simulink model "Sis_Mecanico"  (R2025b)
settings: Solver=VariableStepAuto  StartTime=0.0  StopTime=2  RelTol=1e-3
libraries: fl_lib x7, nesl_utility x3
settings Model: Creator=Brayan Barragan  LastModifiedBy=Brayan Barragan

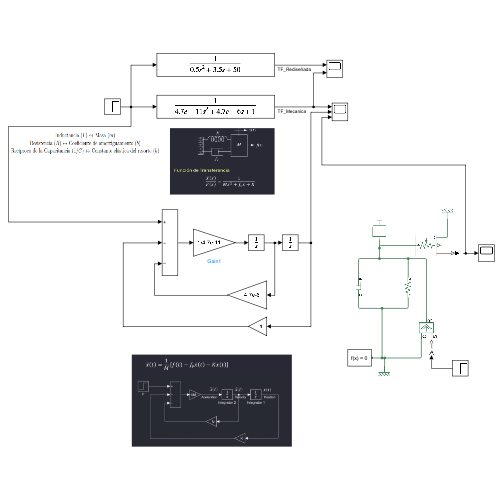
[thumbnail: Simulink's stored preview of the top-level diagram]
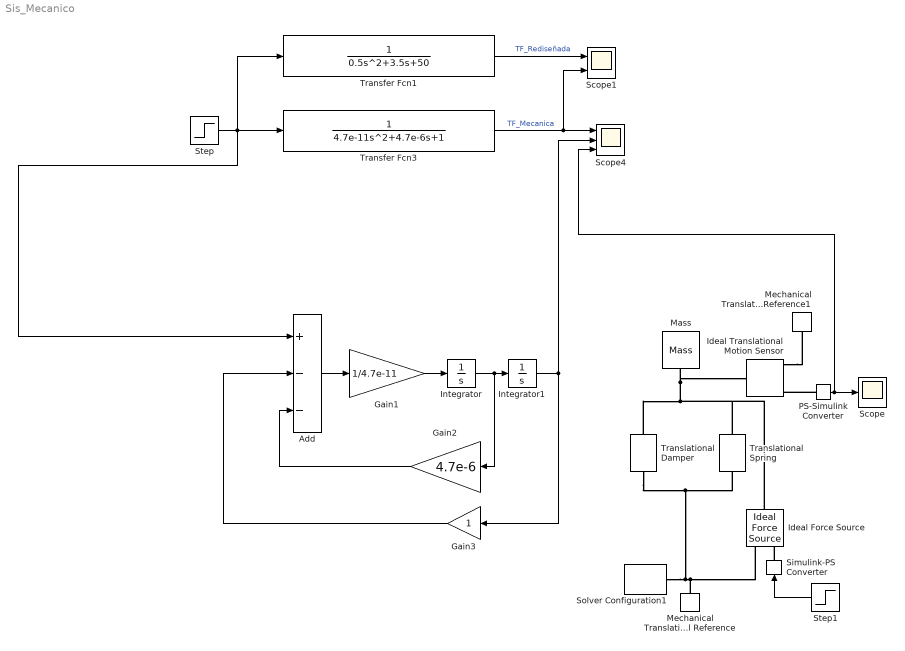
== system Sis_Mecanico ==
  Add : Sum  Inputs=+--
  Gain1 : Gain  Gain=1/4.7e-11
  Gain2 : Gain  Gain=4.7e-6
  Gain3 : Gain
  Ideal Force Source : fl_lib/Mechanical/Mechanical Sources/Ideal Force Source
  Ideal Translational Motion Sensor : fl_lib/Mechanical/Mechanical Sensors/Ideal Translational Motion Sensor  reference=foundation.enum.MeasurementReference.difference  acceleration_port=false  velocity_port=true  position_port=true  offset=0 m
  Integrator : Integrator
  Integrator1 : Integrator
  Mass : fl_lib/Mechanical/Translational Elements/Mass  mass=4.7e-11 kg  num_ports=foundation.enum.numPorts2.one  v_specify=off  v_priority=High  v=0 m/s  v_nominal_specify=off  v_nominal_value=1  v_nominal_unit=m/s  f_specify=off  f_priority=None  f=0 N  f_nominal_specify=off  f_nominal_value=1  f_nominal_unit=N
  Mechanical Translational Reference : fl_lib/Mechanical/Translational Elements/Mechanical Translational Reference
  Mechanical Translational Reference1 : fl_lib/Mechanical/Translational Elements/Mechanical Translational Reference
  PS-Simulink Converter : nesl_utility/PS-Simulink Converter  PhysicalDomain=network_engine_domain  SubClassName=ps_output  LeftPortType=input  RightPortType=output  PseudoPeriodic=off  Frequencies=[]  VectorFormat=inherit  Unit=inherit  AffineConversion=off
  Scope : Scope
      settings: ActiveDisplayYMinimum=-1.6255736050557578E-9  ActiveDisplayYMaximum=1.4630162445501824E-8
  Scope1 : Scope  NumInputPorts=2
      settings: ActiveDisplayYMinimum=-0.0032729739400114018  ActiveDisplayYMaximum=0.029456765460102625
  Scope4 : Scope  NumInputPorts=3
      settings: ActiveDisplayYMinimum=-0.16412239753332028  ActiveDisplayYMaximum=1.4771015777998828  DataLoggingVariableName=ScopeData4
  Simulink-PS Converter : nesl_utility/Simulink-PS Converter  PhysicalDomain=network_engine_domain  SubClassName=ps_input  LeftPortType=input  RightPortType=output  PseudoPeriodic=off  Frequencies=[]  NoiseDistribution=none  NoiseParameters=[]  Unit=1  AffineConversion=off  FilteringAndDerivatives=provide  SimscapeFilterOrder=1  InputFilterTimeConstant=0.001  UdotUserProvided=0
  Solver Configuration1 : nesl_utility/Solver Configuration  PhysicalDomain=network_engine_domain  SubClassName=solver  LeftPortType=input  RightPortType=generic  Tones=[]  Harmonics=[]  SimulateNoise=off  Profile=off  UseLocalSampling=off  EnableSwitchedLinearOptims=on  FrequencyDomain=off  UseCCode=off  RelTol=0.001  AbsTol=0.001  MinStep=1e-09  ToWorkspace=off  RevertToSquareIcSolve=off  NumHomotopyIterations=100  PhasorMode=off  PhasorModeNumHarmonics=1  ConsistencySolver=NEWTON_XTOL_AFTER_FTOL  IndexReductionMethod=DerivativeReplacement  DoDC=off  ResidualTolerance=1e-09  ConsistencyTolSource=GLOBAL  ConsistencyAbsTol=0.001  ConsistencyRelTol=0.001  ConsistencyTolFactor=0.001  UseLocalSolver=off  LocalSolverChoice=NE_BACKWARD_EULER_ADVANCER  ResolveIndetEquations=on  FunctionEvalNumThread=1  LocalSolverSampleTime=0.001  DoFixedCost=off  MaxNonlinIter=3  MaxModeIter=2  ComputeImpulses=off  ImpulseIterations=2  LinearAlgebra=auto  LinearAlgebraNumThread=0  EquationFormulation=NE_TIME_EF  DelaysMemoryBudget=1024  AutomaticFiltering=on  FilteringTimeConstant=0.001  PartitionStorageMethod=AS_NEEDED  PartitionMemoryBudget=1024  PartitionMethod=ROBUST  MultibodyUseLocalSolver=off  MultibodyLocalSolverChoice=ODE1  MultibodyLocalSolverSampleTime=0.001
  Step : Step  SampleTime=0
  Step1 : Step  SampleTime=0
  Transfer Fcn1 : TransferFcn  Denominator=[0.5 3.5 50]
  Transfer Fcn3 : TransferFcn  Denominator=[4.7e-11 4.7e-6 1]
  Translational Damper : fl_lib/Mechanical/Translational Elements/Translational Damper  D=4.7e-6 N*s/m  v_specify=off  v_priority=None  v=0 m/s  v_nominal_specify=off  v_nominal_value=1  v_nominal_unit=m/s  f_specify=off  f_priority=None  f=0 N  f_nominal_specify=off  f_nominal_value=1  f_nominal_unit=N
  Translational Spring : fl_lib/Mechanical/Translational Elements/Translational Spring  spr_rate=1 N/m  v_specify=off  v_priority=None  v=0 m/s  v_nominal_specify=off  v_nominal_value=1  v_nominal_unit=m/s  f_specify=off  f_priority=None  f=0 N  f_nominal_specify=off  f_nominal_value=1  f_nominal_unit=N  x_specify=off  x_priority=High  x=0 m  x_nominal_specify=off  x_nominal_value=1  x_nominal_unit=m
  wires:
  Gain2/1 -> Add/3
  Integrator1/1 -> Scope4/2, Gain3/1
  Gain3/1 -> Add/2
  Integrator/1 -> Gain2/1, Integrator1/1
  Add/1 -> Gain1/1
  Transfer Fcn3/1 -> Scope1/2, Scope4/1  "TF_Mecanica"
  Gain1/1 -> Integrator/1
  Step/1 -> Transfer Fcn1/1, Transfer Fcn3/1, Add/1
  PS-Simulink Converter/1 -> Scope/1, Scope4/3
  Step1/1 -> Simulink-PS Converter/1
  Transfer Fcn1/1 -> Scope1/1  "TF_Rediseñada"
  connections:
  Translational Damper/RConn1 -- Ideal Force Source/RConn2 -- Mechanical Translational Reference/LConn1 -- Solver Configuration1/RConn1 -- Translational Spring/RConn1
  Translational Damper/LConn1 -- Ideal Force Source/LConn1 -- Translational Spring/LConn1 -- Ideal Translational Motion Sensor/LConn1 -- Mass/LConn1
  Ideal Translational Motion Sensor/RConn1 -- Mechanical Translational Reference1/LConn1
  PS-Simulink Converter/LConn1 -- Ideal Translational Motion Sensor/RConn3
  Simulink-PS Converter/RConn1 -- Ideal Force Source/RConn1
